simulink model "NPSS_TTECTrA_PWLM"  (Simulink 7.5)
settings: Solver=ode4  StartTime=0.0  StopTime=60  FixedStep=0.02  RelTol=1e-3
InitFcn:
  | setup_NPSS_Simulink
values from neighbouring files (symbols this model uses):
  A = block.DialogPrm(6).Data    [sfun_xdot2.m]    (also in simFromTTECTrA_PWLM.m = [A lmdata(i).A])
  B = block.DialogPrm(7).Data    [sfun_xdot2.m]    (also in simFromTTECTrA_PWLM.m = [B lmdata(i).B])
  beta = block.DialogPrm(1).Data    [sfun_weights2.m]    (also in simFromTTECTrA_PWLM.m = 25)
  bkpt = block.DialogPrm(1).Data    [sfun_output2.m]    (also in sfun_weights2.m = block.DialogPrm(3).Data; sfun_xdot2.m; simFromTTECTrA_PWLM.m = [bkpt lmdata(i).state(1)])
  bkpt_i = 12    [simFromTTECTrA_PWLM.m]
  C = block.DialogPrm(6).Data    [sfun_output2.m]    (also in simFromTTECTrA_PWLM.m = [C lmdata(i).C])
  D = block.DialogPrm(7).Data    [sfun_output2.m]    (also in simFromTTECTrA_PWLM.m = [D lmdata(i).D])
  mode = block.DialogPrm(2).Data    [sfun_weights2.m]    (also in simFromTTECTrA_PWLM.m = 1)
  x = block.InputPort(1).Data    [sfun_output2.m]    (also in sfun_weights2.m; sfun_xdot2.m; simFromTTECTrA_PWLM.m = [x lmdata(i).state])
  x0 = interp1(u',x',DWS.in.Wf_zro)'    [simFromTTECTrA_PWLM.m]
  y = w(i) * ( y_tr(:,i) + C(:,idx_C)*(x - x_tr(:,i)) + D(:,idx_D)*(u - u_tr(:,i))) + y    [sfun_output2.m]    (also in simFromTTECTrA_PWLM.m = sim(inputs.in.simFileNamePWLM,'SrcWorkspace','base','ReturnW)
undefined symbols (not defined in the file or in its folder): DiscIntNeverNeededParam
libraries: simulink x2
settings Model: Creator=jcsank  LastModifiedBy=jcsank

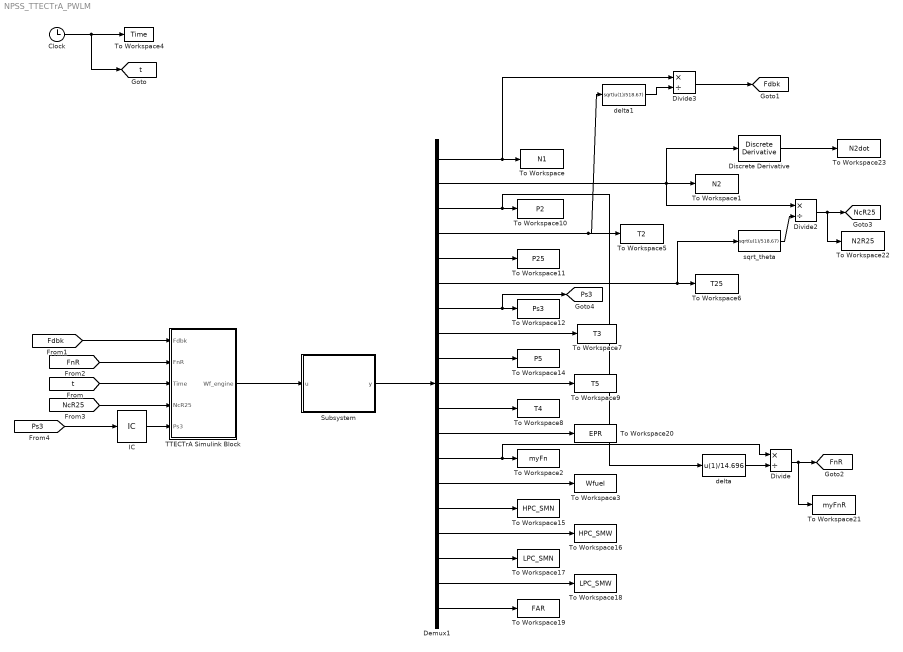
== system NPSS_TTECTrA_PWLM ==
  Clock : Clock
      settings: Decimation=10
  Demux1 : Demux  Outputs=19
  Discrete Derivative : simulink/Discrete/Discrete Derivative  SystemSampleTime=-1  gainval=1.0  ICPrevScaledInput=0.0  OutMin=[]  OutMax=[]  OutDataType=fixdt(1, 16)  OutScaling=2^-10  DoSatur=off
  Divide : Product  Inputs=*/
  Divide2 : Product  Inputs=*/
  Divide3 : Product  Inputs=*/
  IC : InitialCondition  Value=5000
  Subsystem : Subsystem
  TTECTrA Simulink Block : Subsystem
  To Workspace : ToWorkspace  VariableName=N1  SampleTime=-1  SaveFormat=Array
  To Workspace1 : ToWorkspace  VariableName=N2  SampleTime=-1  SaveFormat=Array
  To Workspace10 : ToWorkspace  VariableName=P2  SampleTime=-1  SaveFormat=Array
  To Workspace11 : ToWorkspace  VariableName=P25  SampleTime=-1  SaveFormat=Array
  To Workspace12 : ToWorkspace  VariableName=Ps3  SampleTime=-1  SaveFormat=Array
  To Workspace14 : ToWorkspace  VariableName=P5  SampleTime=-1  SaveFormat=Array
  To Workspace15 : ToWorkspace  VariableName=HPC_SMN  SampleTime=-1  SaveFormat=Array
  To Workspace16 : ToWorkspace  VariableName=HPC_SMW  SampleTime=-1  SaveFormat=Array
  To Workspace17 : ToWorkspace  VariableName=LPC_SMN  SampleTime=-1  SaveFormat=Array
  To Workspace18 : ToWorkspace  VariableName=LPC_SMW  SampleTime=-1  SaveFormat=Array
  To Workspace19 : ToWorkspace  VariableName=FAR  SampleTime=-1  SaveFormat=Array
  To Workspace2 : ToWorkspace  VariableName=myFn  SampleTime=-1  SaveFormat=Array
  To Workspace20 : ToWorkspace  VariableName=EPR  SampleTime=-1  SaveFormat=Array
  To Workspace21 : ToWorkspace  VariableName=myFnR  SampleTime=-1  SaveFormat=Array
  To Workspace22 : ToWorkspace  VariableName=N2R25  SampleTime=-1  SaveFormat=Array
  To Workspace23 : ToWorkspace  VariableName=N2dot  SampleTime=-1  SaveFormat=Array
  To Workspace3 : ToWorkspace  VariableName=Wfuel  SampleTime=-1  SaveFormat=Array
  To Workspace4 : ToWorkspace  VariableName=Time  SampleTime=-1  SaveFormat=Array
  To Workspace5 : ToWorkspace  VariableName=T2  SampleTime=-1  SaveFormat=Array
  To Workspace6 : ToWorkspace  VariableName=T25  SampleTime=-1  SaveFormat=Array
  To Workspace7 : ToWorkspace  VariableName=T3  SampleTime=-1  SaveFormat=Array
  To Workspace8 : ToWorkspace  VariableName=T4  SampleTime=-1  SaveFormat=Array
  To Workspace9 : ToWorkspace  VariableName=T5  SampleTime=-1  SaveFormat=Array
  delta : Fcn  Expr=u(1)/14.696
  delta1 : Fcn  Expr=sqrt(u(1)/518.67)
  sqrt_theta : Fcn  Expr=sqrt(u(1)/518.67)
  tag scope: Fdbk=global, FnR=global, NcR25=global, Ps3=global, t=global
  wires:
  Subsystem/1(y) -> Demux1/1
  Clock/1 -> [t], To Workspace4/1
  TTECTrA Simulink Block/1(Wf_engine) -> Subsystem/1(u)
  [t] -> TTECTrA Simulink Block/3(Time)
  [Fdbk] -> TTECTrA Simulink Block/1(Fdbk)
  [FnR] -> TTECTrA Simulink Block/2("FnR ")
  [NcR25] -> TTECTrA Simulink Block/4(NcR25)
  Divide/1 -> [FnR], To Workspace21/1
  delta/1 -> Divide/2
  Divide2/1 -> [NcR25], To Workspace22/1
  Discrete Derivative/1 -> To Workspace23/1
  [Ps3] -> IC/1
  IC/1 -> TTECTrA Simulink Block/5(Ps3)
  Demux1/1 -> To Workspace/1, Divide3/1
  Demux1/2 -> To Workspace1/1, Discrete Derivative/1, Divide2/1
  Demux1/3 -> To Workspace10/1, delta/1
  Demux1/4 -> To Workspace5/1, delta1/1
  Demux1/5 -> To Workspace11/1
  Demux1/6 -> To Workspace6/1, sqrt_theta/1
  Demux1/7 -> To Workspace12/1, [Ps3]
  Demux1/8 -> To Workspace7/1
  Demux1/10 -> To Workspace9/1
  Demux1/9 -> To Workspace14/1
  Demux1/11 -> To Workspace8/1
  Demux1/12 -> To Workspace20/1
  Demux1/13 -> To Workspace2/1, Divide/1
  Demux1/14 -> To Workspace3/1
  Demux1/15 -> To Workspace15/1
  Demux1/16 -> To Workspace16/1
  Demux1/17 -> To Workspace17/1
  Demux1/18 -> To Workspace18/1
  Demux1/19 -> To Workspace19/1
  sqrt_theta/1 -> Divide2/2
  delta1/1 -> Divide3/2
  Divide3/1 -> [Fdbk]

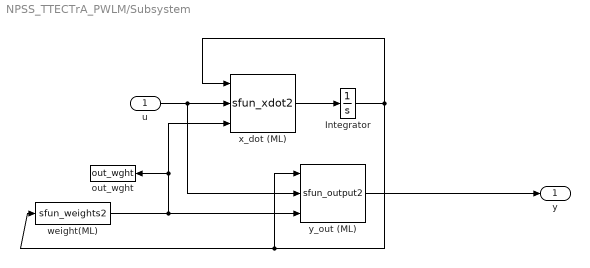
== system NPSS_TTECTrA_PWLM/Subsystem ==
  u : Inport  OutDataType=fixdt(1, 16)  OutScaling=2^0
  Integrator : Integrator  InitialCondition=x0
  out_wght : ToWorkspace  VariableName=out_wght  SampleTime=-1  SaveFormat=Array
  "weight(ML) " : M-S-Function  FunctionName=sfun_weights2  Parameters=beta,mode,bkpt,bkpt_i,x,y
  x_dot (ML) : M-S-Function  FunctionName=sfun_xdot2  Parameters=bkpt,bkpt_i,x,u,y,A,B
  y_out (ML) : M-S-Function  FunctionName=sfun_output2  Parameters=bkpt,bkpt_i,x,u,y,C,D
  y : Outport  OutDataType=fixdt(1, 16)  OutScaling=2^0
  wires:
  u/1 -> y_out (ML)/2, x_dot (ML)/2
  x_dot (ML)/1 -> Integrator/1
  Integrator/1 -> y_out (ML)/1, "weight(ML) "/1, x_dot (ML)/1
  "weight(ML) "/1 -> y_out (ML)/3, out_wght/1, x_dot (ML)/3
  y_out (ML)/1 -> y/1

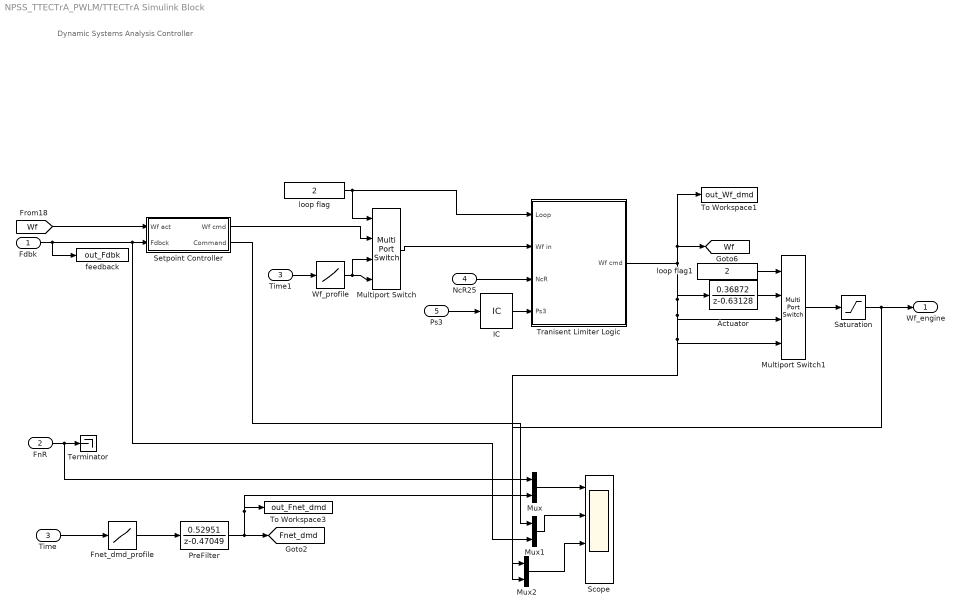
== system NPSS_TTECTrA_PWLM/TTECTrA Simulink Block ==
  note: Dynamic Systems Analysis Controller
  Fdbk : Inport
  "FnR " : Inport  Port=2
  Time : Inport  Port=3
  NcR25 : Inport  Port=4
  Ps3 : Inport  Port=5
  Actuator : DiscreteTransferFcn  Numerator=[0.36872]  Denominator="[1    -0.63128]"  SampleTime=-1
  Fnet_dmd_profile : Lookup  InputValues="[0  10  15  20  30  35]"  Table="[30000  30000  30000  30000  30000  30000]"  SampleTime=0.02
  IC : InitialCondition
  Multiport Switch : MultiPortSwitch  zeroidx=off  SampleTime=0.02
  Multiport Switch1 : MultiPortSwitch  zeroidx=off  SampleTime=0.02
  Mux : Mux  Inputs=2
  Mux1 : Mux  Inputs=2
  Mux2 : Mux  Inputs=2
  PreFilter : DiscreteTransferFcn  Numerator=[0.52951]  Denominator="[1    -0.47049]"  SampleTime=-1
  Saturation : Saturate  UpperLimit=9999  LowerLimit=0
  Scope : Scope  NumInputPorts=4
      settings: TimeRange=20  YMin=0~0~0.353058~-1  YMax=30000~30000~0.390222~1
  Setpoint Controller : Subsystem
  Terminator : Terminator
  Time1 : InportShadow  Port=3
  To Workspace1 : ToWorkspace  VariableName=out_Wf_dmd  SampleTime=-1  SaveFormat=Array
  To Workspace3 : ToWorkspace  VariableName=out_Fnet_dmd  SampleTime=-1  SaveFormat=Array
  Tranisent Limiter Logic : Subsystem
  Wf_profile : Lookup  InputValues="[0  10  15  20  30  35]"  Table="[0.53679     0.53679      2.5797      2.5797     0.53679     0.53679]"  SampleTime=0.02
  feedback : ToWorkspace  VariableName=out_Fdbk  SampleTime=-1  SaveFormat=Array
  loop flag : Constant  Value=2
  loop flag1 : Constant  Value=2
  Wf_engine : Outport
  tag scope: Fnet_dmd=global, Wf=global
  wires:
  [Wf] -> Setpoint Controller/1(Wf act)
  Fdbk/1 -> feedback/1, Setpoint Controller/2(Fdbck), Mux1/2
  Time/1 -> Fnet_dmd_profile/1
  NcR25/1 -> Tranisent Limiter Logic/3(NcR)
  Fnet_dmd_profile/1 -> PreFilter/1
  PreFilter/1 -> [Fnet_dmd], To Workspace3/1, Mux/2
  Saturation/1 -> Wf_engine/1, Mux2/1
  Multiport Switch1/1 -> Saturation/1
  loop flag1/1 -> Multiport Switch1/1
  Ps3/1 -> IC/1
  Time1/1 -> Wf_profile/1
  loop flag/1 -> Tranisent Limiter Logic/1(Loop), Multiport Switch/1
  Multiport Switch/1 -> Tranisent Limiter Logic/2(Wf in)
  Wf_profile/1 -> Multiport Switch/4, Multiport Switch/3
  Setpoint Controller/1(Wf cmd) -> Multiport Switch/2
  IC/1 -> Tranisent Limiter Logic/4(Ps3)
  "FnR "/1 -> Terminator/1, Mux/1
  Mux/1 -> Scope/1
  Mux1/1 -> Scope/2
  Setpoint Controller/2(Command) -> Mux1/1
  Mux2/1 -> Scope/3
  Actuator/1 -> Multiport Switch1/2
  Tranisent Limiter Logic/1(Wf cmd) -> [Wf], To Workspace1/1, Multiport Switch1/3, Multiport Switch1/4, Mux2/2, Actuator/1

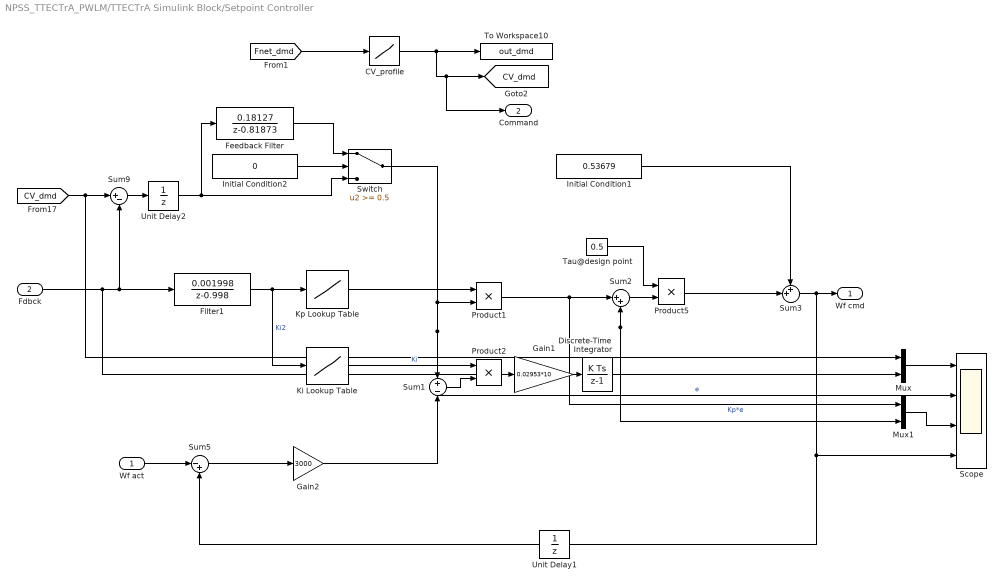
== system NPSS_TTECTrA_PWLM/TTECTrA Simulink Block/Setpoint Controller ==
  Wf act : Inport
  Fdbck : Inport  Port=2
  CV_profile : Lookup  InputValues="[1  2]"  Table="[1  2]"  LookUpMeth=Interpolation-Use End Values  SampleTime=0.02
  Discrete-Time Integrator : DiscreteIntegrator  SampleTime=-1  ICPrevOutput=DiscIntNeverNeededParam  ICPrevScaledInput=DiscIntNeverNeededParam
  Feedback Filter : DiscreteTransferFcn  Numerator=[0.18127]  Denominator="[1    -0.81873]"  SampleTime=0.02
  Filter1 : DiscreteTransferFcn  Numerator=[0.001998]  Denominator="[1      -0.998]"  SampleTime=0.02
  Gain1 : Gain  Gain=0.02953*10
  Gain2 : Gain  Gain=3000
  Initial Condition1 : Constant  Value=0.53679
  Initial Condition2 : Constant  Value=0
  Ki Lookup Table : Lookup_n-D  NumberOfTableDimensions=1  BreakpointsForDimension1="[1000  5000]"  Table="[1  2]"  SampleTime=0.02  RndMeth=Simplest  InputSameDT=on
  Kp Lookup Table : Lookup_n-D  NumberOfTableDimensions=1  BreakpointsForDimension1="[1000  5000]"  Table="[1  2]"  SampleTime=0.02  RndMeth=Simplest  InputSameDT=on
  Mux : Mux  Inputs=2
  Mux1 : Mux  Inputs=2
  Product1 : Product  SampleTime=0.02  RndMeth=Zero
  Product2 : Product  RndMeth=Zero
  Product5 : Product  SampleTime=0.02  RndMeth=Zero
  Scope : Scope  NumInputPorts=4
      settings: TimeRange=15  YMin=500~4305~-10~0.34  YMax=5500~4319~10~0.43
  Sum1 : Sum  Inputs=+|-
  Sum2 : Sum  Inputs=|++  SampleTime=0.02
  Sum3 : Sum  Inputs=++|  SampleTime=0.02
  Sum5 : Sum  Inputs=|-+
  Sum9 : Sum  Inputs=|+-  SampleTime=0.02
  Switch : Switch  Threshold=0.5  SampleTime=0.02
  Tau@design point : Constant  Value=0.5
  To Workspace10 : ToWorkspace  VariableName=out_dmd  SampleTime=-1  SaveFormat=Array
  Unit Delay1 : UnitDelay  SampleTime=-1
  Unit Delay2 : UnitDelay  SampleTime=-1
  Wf cmd : Outport
  Command : Outport  Port=2
  tag scope: CV_dmd=global
  wires:
  Tau@design point/1 -> Product5/1
  Product1/1 -> Sum2/1, Mux1/1  "Kp*e"
  Product2/1 -> Gain1/1
  Sum9/1 -> Unit Delay2/1
  [CV_dmd] -> Sum9/1, Mux/1
  Wf act/1 -> Sum5/1
  Sum5/1 -> Gain2/1
  Switch/1 -> Product1/2, Sum1/1, Scope/2  "e"
  Sum1/1 -> Product2/2
  Sum2/1 -> Product5/2
  Gain2/1 -> Sum1/2
  Sum3/1 -> Wf cmd/1, Unit Delay1/1, Scope/4
  Initial Condition1/1 -> Sum3/1
  Product5/1 -> Sum3/2
  Gain1/1 -> Discrete-Time Integrator/1
  Discrete-Time Integrator/1 -> Sum2/2, Mux1/2
  Ki Lookup Table/1 -> Product2/1  "Ki"
  Fdbck/1 -> Sum9/2, Filter1/1, Mux/2
  CV_profile/1 -> To Workspace10/1, [CV_dmd], Command/1
  [Fnet_dmd] -> CV_profile/1
  Kp Lookup Table/1 -> Product1/1
  Filter1/1 -> Ki Lookup Table/1, Kp Lookup Table/1  "Ki2"
  Initial Condition2/1 -> Switch/2
  Feedback Filter/1 -> Switch/1
  Unit Delay1/1 -> Sum5/2
  Mux/1 -> Scope/1
  Mux1/1 -> Scope/3
  Unit Delay2/1 -> Switch/3, Feedback Filter/1

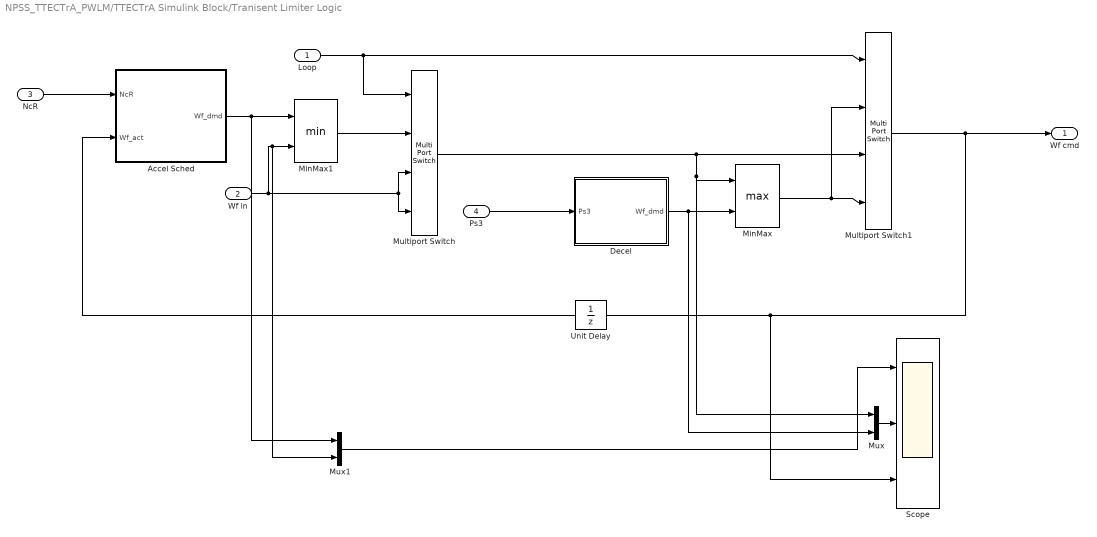
== system NPSS_TTECTrA_PWLM/TTECTrA Simulink Block/Tranisent Limiter Logic ==
  Loop : Inport
  Wf in : Inport  Port=2
  NcR : Inport  Port=3
  Ps3 : Inport  Port=4
  Accel Sched : Subsystem
  Decel : Subsystem
  MinMax : MinMax  Function=max  Inputs=2  SampleTime=0.02
  MinMax1 : MinMax  Inputs=2  SampleTime=0.02
  Multiport Switch : MultiPortSwitch  zeroidx=off  SampleTime=0.02
  Multiport Switch1 : MultiPortSwitch  zeroidx=off  SampleTime=0.02
  Mux : Mux  Inputs=2
  Mux1 : Mux  Inputs=2
  Scope : Scope  NumInputPorts=3
      settings: TimeRange=60  YMin=-1~-1~5.55112e-017  YMax=10~1~0.9  SaveName=ScopeData2
  Unit Delay : UnitDelay  SampleTime=-1
  Wf cmd : Outport
  wires:
  NcR/1 -> Accel Sched/1(NcR)
  Unit Delay/1 -> Accel Sched/2(Wf_act)
  Loop/1 -> Multiport Switch/1, Multiport Switch1/1
  Accel Sched/1(Wf_dmd) -> Mux1/1, MinMax1/1
  Wf in/1 -> MinMax1/2, Mux1/2, Multiport Switch/4, Multiport Switch/3
  Ps3/1 -> Decel/1(Ps3)
  Multiport Switch1/1 -> Wf cmd/1, Unit Delay/1, Scope/3
  MinMax/1 -> Multiport Switch1/4, Multiport Switch1/2
  Multiport Switch/1 -> Multiport Switch1/3, MinMax/1, Mux/1
  Decel/1(Wf_dmd) -> MinMax/2, Mux/2
  Mux/1 -> Scope/2
  Mux1/1 -> Scope/1
  MinMax1/1 -> Multiport Switch/2

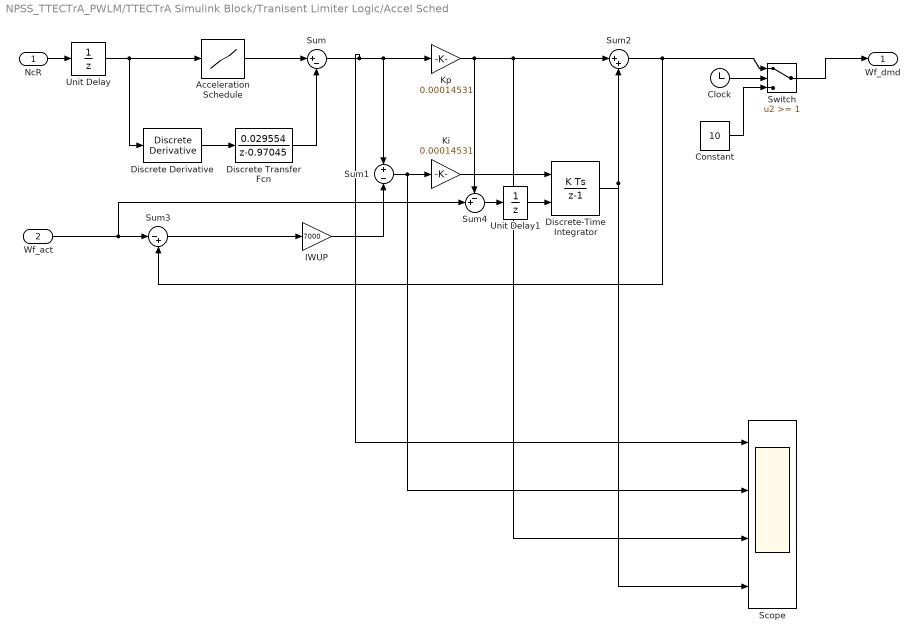
== system NPSS_TTECTrA_PWLM/TTECTrA Simulink Block/Tranisent Limiter Logic/Accel Sched ==
  NcR : Inport
  Wf_act : Inport  Port=2
  Acceleration Schedule : Lookup  InputValues="[7500  11000]"  Table="[150  150]"  SampleTime=0.02
  Clock : Clock
      settings: Decimation=10
  Constant : Constant  Value=10  OutDataType=fixdt(1, 16)  OutScaling=2^0
  Discrete Derivative : simulink/Discrete/Discrete Derivative  SystemSampleTime=-1  gainval=1.0  ICPrevScaledInput=0  OutMin=[]  OutMax=[]  OutDataType=fixdt(1, 16)  OutScaling=2^-10  DoSatur=off
  Discrete Transfer Fcn : DiscreteTransferFcn  Numerator=[0.029554]  Denominator="[1    -0.97045]"  SampleTime=0.02
  Discrete-Time Integrator : DiscreteIntegrator  InitialConditionSource=external  SampleTime=0.02  ICPrevOutput=DiscIntNeverNeededParam  ICPrevScaledInput=DiscIntNeverNeededParam
  IWUP : Gain  Gain=7000
  Ki : Gain  Gain=0.00014531
  Kp : Gain  Gain=0.00014531  SampleTime=0.02
  Scope : Scope  NumInputPorts=4
      settings: YMin=590.006~547.139~0.0857338~-1  YMax=590.006~547.139~0.0857338~1  SaveName=ScopeData5
  Sum : Sum  Inputs=|+-  SampleTime=0.02
  Sum1 : Sum  Inputs=+|-
  Sum2 : Sum  Inputs=|++  SampleTime=0.02
  Sum3 : Sum  Inputs=|-+
  Sum4 : Sum  Inputs=-+|  SampleTime=0.02
  Switch : Switch  Threshold=1  OutDataType=fixdt(1, 16)  OutScaling=2^0
  Unit Delay : UnitDelay  SampleTime=-1
  Unit Delay1 : UnitDelay  SampleTime=-1
  Wf_dmd : Outport
  wires:
  NcR/1 -> Unit Delay/1
  Discrete Derivative/1 -> Discrete Transfer Fcn/1
  Acceleration Schedule/1 -> Sum/1
  Discrete Transfer Fcn/1 -> Sum/2
  Sum/1 -> Sum1/1, Kp/1, Scope/1
  Sum1/1 -> Ki/1, Scope/2
  Kp/1 -> Sum4/1, Sum2/1, Scope/3
  Sum2/1 -> Sum3/2, Switch/1
  Ki/1 -> Discrete-Time Integrator/1
  Discrete-Time Integrator/1 -> Sum2/2, Scope/4
  IWUP/1 -> Sum1/2
  Sum3/1 -> IWUP/1
  Wf_act/1 -> Sum4/2, Sum3/1
  Sum4/1 -> Unit Delay1/1
  Unit Delay/1 -> Discrete Derivative/1, Acceleration Schedule/1
  Unit Delay1/1 -> Discrete-Time Integrator/2
  Clock/1 -> Switch/2
  Constant/1 -> Switch/3
  Switch/1 -> Wf_dmd/1

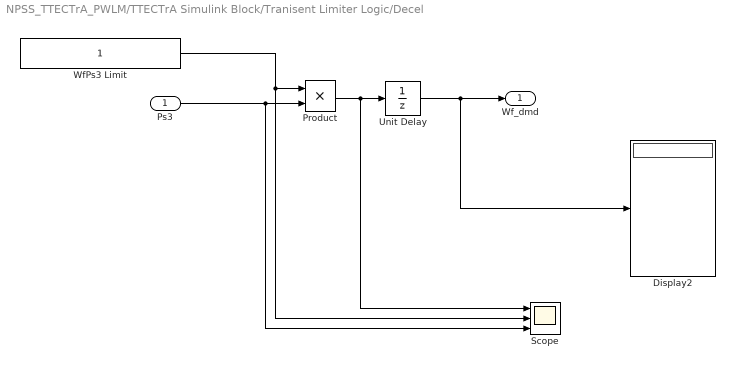
== system NPSS_TTECTrA_PWLM/TTECTrA Simulink Block/Tranisent Limiter Logic/Decel ==
  Ps3 : Inport
  Display2 : Display
  Product : Product  RndMeth=Zero
  Scope : Scope  NumInputPorts=3
      settings: YMin=-5~-5~-5  YMax=5~5~5  SaveName=ScopeData4
  Unit Delay : UnitDelay  X0=0.53679  SampleTime=-1
  WfPs3 Limit : Constant
  Wf_dmd : Outport
  wires:
  Ps3/1 -> Product/2, Scope/3
  WfPs3 Limit/1 -> Product/1, Scope/2
  Product/1 -> Unit Delay/1, Scope/1
  Unit Delay/1 -> Wf_dmd/1, Display2/1
